simulink model "test_b_computing_dt"  (R2020b)
settings: Solver=FixedStepAuto  StartTime=0.0  StopTime=6  FixedStep=0.01  RelTol=1e-3
settings Model: Creator=kika  LastModifiedBy=kika

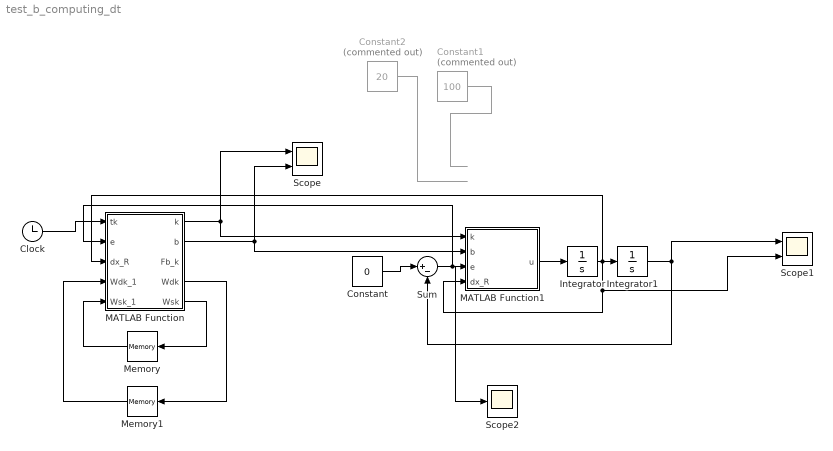
== system test_b_computing_dt ==
  Clock : Clock
  Constant : Constant  Value=0
  Constant1 : Constant  Commented=on  Value=100
  Constant2 : Constant  Commented=on  Value=20
  Integrator : Integrator  InitialCondition=1
  Integrator1 : Integrator  InitialCondition=1
  MATLAB Function : MATLAB Function  TreatAsAtomicUnit=on
  MATLAB Function1 : MATLAB Function  TreatAsAtomicUnit=on
  Memory : Memory
  Memory1 : Memory
  Scope : Scope  NumInputPorts=2
  Scope1 : Scope  NumInputPorts=2
  Scope2 : Scope
  Sum : Sum  Inputs=|+-
  wires:
  Clock/1 -> MATLAB Function/1(tk)
  MATLAB Function/5(Wsk) -> Memory/1
  Memory/1 -> MATLAB Function/5(Wsk_1)
  MATLAB Function/4(Wdk) -> Memory1/1
  Memory1/1 -> MATLAB Function/4(Wdk_1)
  MATLAB Function/1(k) -> MATLAB Function1/1(k), Scope/1
  MATLAB Function/2(b) -> MATLAB Function1/2(b), Scope/2
  Integrator/1 -> Scope1/2, MATLAB Function1/4(dx_R), MATLAB Function/3(dx_R), Integrator1/1
  Sum/1 -> Scope2/1, MATLAB Function/2(e), MATLAB Function1/3(e)
  MATLAB Function1/1(u) -> Integrator/1
  Integrator1/1 -> Sum/2, Scope1/1
  Constant/1 -> Sum/1
  Constant2/1 -> ?
  Constant1/1 -> ?

== matlab function test_b_computing_dt/MATLAB Function1 ==
  data: k input; u output; b input; e input; dx_R input
function u = fcn(k, b, e, dx_R)

    u = k*e - b*dx_R;

== matlab function test_b_computing_dt/MATLAB Function ==
  data: tk input; e input; dx_R input; k output; b output; Fb_k output; Wdk output; Wsk output; Wdk_1 input; Wsk_1 input
function [k, b, Fb_k, Wdk, Wsk] = fcn(tk, e, dx_R, Wdk_1, Wsk_1)

    DeltaEtot = 0.5 * 1 * 1^2 + 0.5 * 1 * 0^2;
    T_R = 0.01;
    
    k = -2*tk + 10;
    
    
    b =  -(DeltaEtot + Wdk_1 + Wsk_1 + k * e *dx_R* T_R) / (dx_R^2 * T_R) + 3;
    
    Fb_k = b * dx_R;
    Wdk = Wdk_1 + Fb_k * dx_R * T_R;
    Wsk = Wsk_1 + k * e * dx_R * T_R;
